simulink library "Quaternion_Subtraction"  (R2016a)
settings: Solver=ode45  StartTime=0.0  StopTime=10.0  RelTol=1e-3
libraries: Quaternion_Conjugate x1, Quaternion_Multiplication x1
settings Model: Creator=devantormey  LastModifiedBy=devantormey
settings DataIOCC: LimitDataPoints=on
settings DebuggingCC: AllowSymbolicDim=off

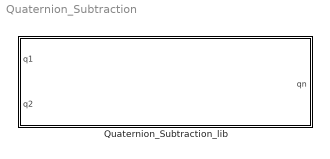
== system Quaternion_Subtraction ==
  Quaternion_Subtraction_lib : Subsystem

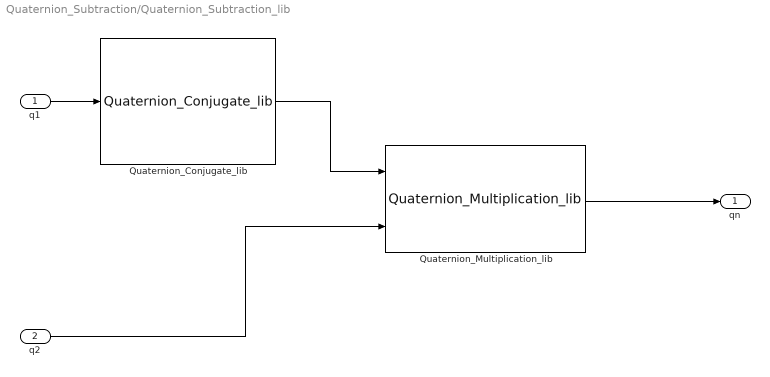
== system Quaternion_Subtraction/Quaternion_Subtraction_lib ==
  q1 : Inport
  q2 : Inport  Port=2
  Quaternion_Conjugate_lib : Quaternion_Conjugate/Quaternion_Conjugate_lib
  Quaternion_Multiplication_lib : Quaternion_Multiplication/Quaternion_Multiplication_lib
  qn : Outport
  wires:
  Quaternion_Multiplication_lib/1 -> qn/1
  Quaternion_Conjugate_lib/1 -> Quaternion_Multiplication_lib/1
  q1/1 -> Quaternion_Conjugate_lib/1
  q2/1 -> Quaternion_Multiplication_lib/2
